simulink model "Experiment_cs"  (Simulink 8.8)
settings: Solver=ode5  StartTime=0.0  StopTime=inf  FixedStep=0.0005  RelTol=1e-3
PreLoadFcn:
  | check_NUTS_defined;
  | 
  | assignin('base',['model_closed_' bdroot],false);
InitFcn:
  | PreScanExperimentInitFcn(bdroot)
StopFcn:
  | PreScanExperimentStopFcn(bdroot)
undefined symbols (not defined in the file): DiscIntNeverNeededParam, FromPrescan, IdealSensors, psi, vd01, vd02, vd03, vd4, x, y
libraries: PreScanSimulinkLibrary x12, PreScanUsefulBlocks x8
(part 3 of 5)

== system Experiment_cs/Mazda_RX8_1/Dynamics_UserSpecified/SingleVehicle_01/VehicleDynamics ==
  VehicleStateLast : Inport
  accelCmd : Inport  Port=2
  brakeCmd : Inport  Port=3
  steerCmd : Inport  Port=4
  Bus Assignment : BusAssignment  AssignedSignals=x,y,psi
  Bus Selector : BusSelector  OutputSignals=x,y,z,u,v,w,theta,phi,psi
  F by m : Gain  Gain=1/veh_struct.mass*1000
  Integrator : Integrator  InitialCondition=veh_struct.init.u
  KinematicVehicleModel : MATLAB Function  TreatAsAtomicUnit=on
  MuxState : Subsystem  Tag=MuxState  mask(Empty Dynamics State Block){positioningmode=on, TimeStep=1/20}
      mask prompts: positioningmode "Positioning Mode"; TimeStep "Auto Assigned: Time Step [s]"
      mask help:
      | Build the state of an actor based on user input.
      | The user can either use positioning mode or dynamics mode.
      | - When using positioning mode the position and orientation of the actor are set directly based on the input. Expected input is relative to the initial position and orientation of the actor. It's also possible to specify the velocity of the actor, though this input isn't used, only passed on.
      | - When using dynamics mode the position input is ignored. Expected input is velocity and orientation. The velocity is relative the current orientation of the actor, while orientation is relative to its initial orientation. The position of the actor is calculated based on the velocity and orientation given.
      settings: DeleteFcn=PreScanBlockDeleteFcn;
  Scope : Scope
  Sum : Sum  Inputs=|++
  int_dX : Integrator  InitialCondition=veh_struct.init.X
  int_dY : Integrator  InitialCondition=veh_struct.init.Y
  int_dpsi : Integrator  InitialCondition=veh_struct.init.psi
  VehicleStateBus : Outport
  PrescanState : Outport  Port=2
  wires:
  int_dpsi/1 -> KinematicVehicleModel/3(psi), Bus Assignment/4
  int_dY/1 -> Bus Assignment/3
  int_dX/1 -> Bus Assignment/2
  KinematicVehicleModel/3(dpsi) -> int_dpsi/1
  KinematicVehicleModel/1(dX) -> int_dX/1
  KinematicVehicleModel/2(dY) -> int_dY/1
  Integrator/1 -> KinematicVehicleModel/1(u), Scope/1
  F by m/1 -> Integrator/1
  Sum/1 -> F by m/1
  brakeCmd/1 -> Sum/2
  accelCmd/1 -> Sum/1
  steerCmd/1 -> KinematicVehicleModel/2(delta)
  VehicleStateLast/1 -> Bus Assignment/1
  Bus Selector/8 -> MuxState/8(P [rad])  "<phi>"
  Bus Selector/9 -> MuxState/9(Y [rad])  "<psi>"
  Bus Selector/7 -> MuxState/7(R [rad])  "<theta>"
  Bus Selector/2 -> MuxState/2(y [m])  "<y>"
  Bus Selector/1 -> MuxState/1(x [m])  "<x>"
  Bus Selector/6 -> MuxState/6(dz [m/s])  "<w>"
  Bus Selector/5 -> MuxState/5(dy [m/s])  "<v>"
  Bus Selector/4 -> MuxState/4(dx [m/s])  "<u>"
  Bus Selector/3 -> MuxState/3(z [m])  "<z>"
  Bus Assignment/1 -> VehicleStateBus/1, Bus Selector/1
  MuxState/1(state) -> PrescanState/1

== system Experiment_cs/Mazda_RX8_1/SELF_Demux/compas converter/cart2compas ==
  Angle [deg] : Inport
  Constant : Constant  Value=90
  Constant1 : Constant  Value=360
  Gain : Gain  Gain=1/360
  Gain1 : Gain  Gain=360
  Gain2 : Gain  Gain=-1
  Rounding Function : Rounding
  Sum : Sum  Inputs=|-+
  Sum1 : Sum  Inputs=-+|
  Sum2 : Sum  Inputs=++|
  heading [deg] : Outport
  wires:
  Sum2/1 -> heading [deg]/1
  Constant1/1 -> Sum2/1
  Gain2/1 -> Sum2/2
  Constant/1 -> Sum1/1
  Sum1/1 -> Sum/2, Gain/1
  Sum/1 -> Gain2/1
  Angle [deg]/1 -> Sum1/2
  Gain1/1 -> Sum/1
  Rounding Function/1 -> Gain1/1
  Gain/1 -> Rounding Function/1

== system Experiment_cs/Toyota_Yaris_1/Dynamics_UserSpecified/SingleVehicle_01/Controller ==
  VehcileStateLast : Inport
  PrescanSimData : Inport  Port=2
  Trigger : TriggerPort  VariantControl=Variant  PortDimensions=1
  Actuation : Subsystem
  CollectSensorData : Subsystem
  CtlMainBusUnitDelayAndInit : Subsystem
  FeaturedFunctions : Subsystem
  SituationalAwareness : Subsystem
  StrategicArbitration : Subsystem
  accelCmd : Outport
  brakeCmd : Outport  Port=2
  steerCmd : Outport  Port=3
  ControllerMainBus : Outport  Port=4
  wires:
  CollectSensorData/2(IdealSensorBus) -> SituationalAwareness/2(IdealSensorBus)
  CollectSensorData/1(PrescanSimDataBus) -> SituationalAwareness/1(PrescanSimDataBus)
  CtlMainBusUnitDelayAndInit/1(CtlBusDelayed) -> CollectSensorData/3(ControllerMainBusIn)
  Actuation/4(ControllerMainBusOut) -> ControllerMainBus/1, CtlMainBusUnitDelayAndInit/1(CtlBus)
  VehcileStateLast/1 -> CollectSensorData/2(VehicleStateLast)
  CollectSensorData/3(ControllerMainBusOut) -> SituationalAwareness/3(ControllerMainBusIn)
  SituationalAwareness/2(ControllerMainBusOut) -> FeaturedFunctions/2(ControllerMainBusIn)
  SituationalAwareness/1(SituationBus) -> FeaturedFunctions/1(SituationBus)
  FeaturedFunctions/1(FeatureReqBus) -> StrategicArbitration/1(FeatureReqBus)
  FeaturedFunctions/2(ControllerMainBusOut) -> StrategicArbitration/2(ControllerMainBusIn)
  StrategicArbitration/2(ControllerMainBusOut) -> Actuation/2(ControllerMainBusIn)
  StrategicArbitration/1(ArbitratedActuationReq) -> Actuation/1(ArbitratedActuationReq)
  Actuation/3(steerCmd) -> steerCmd/1
  Actuation/2(brakeCmd) -> brakeCmd/1
  Actuation/1(accelCmd) -> accelCmd/1
  PrescanSimData/1 -> CollectSensorData/1(PreScanSimData)

== system Experiment_cs/Toyota_Yaris_1/Dynamics_UserSpecified/SingleVehicle_01/Monitor ==
  VehicleStateBus : Inport
  ControllerMainBus : Inport  Port=2
  ControllerMainBusStorage : Subsystem
  VehicleStateBusStorage : ToWorkspace  VariableName=vd02_DataVehicleBus  SaveFormat=Timeseries  SampleTime=-1
  wires:
  ControllerMainBus/1 -> ControllerMainBusStorage/1(ControllerMainBus)
  VehicleStateBus/1 -> VehicleStateBusStorage/1

== system Experiment_cs/Toyota_Yaris_1/Dynamics_UserSpecified/SingleVehicle_01/VehStateBusUnitDelayAndInit ==
  VehStateBus : Inport
  MATLAB Function : MATLAB Function  TreatAsAtomicUnit=on
  Memory : Memory  InheritSampleTime=on
  VehStateBusDelayed : Outport
  wires:
  MATLAB Function/1(y) -> VehStateBusDelayed/1
  VehStateBus/1 -> Memory/1
  Memory/1 -> MATLAB Function/1(u)

== system Experiment_cs/Toyota_Yaris_1/Dynamics_UserSpecified/SingleVehicle_01/VehicleDynamics ==
  VehicleStateLast : Inport
  accelCmd : Inport  Port=2
  brakeCmd : Inport  Port=3
  steerCmd : Inport  Port=4
  Bus Assignment : BusAssignment  AssignedSignals=x,y,psi
  Bus Selector : BusSelector  OutputSignals=x,y,z,u,v,w,theta,phi,psi
  F by m : Gain  Gain=1/veh_struct.mass*1000
  Integrator : Integrator  InitialCondition=veh_struct.init.u
  KinematicVehicleModel : MATLAB Function  TreatAsAtomicUnit=on
  MuxState : Subsystem  Tag=MuxState  mask(Empty Dynamics State Block){positioningmode=on, TimeStep=1/20}
      mask prompts: positioningmode "Positioning Mode"; TimeStep "Auto Assigned: Time Step [s]"
      mask help:
      | Build the state of an actor based on user input.
      | The user can either use positioning mode or dynamics mode.
      | - When using positioning mode the position and orientation of the actor are set directly based on the input. Expected input is relative to the initial position and orientation of the actor. It's also possible to specify the velocity of the actor, though this input isn't used, only passed on.
      | - When using dynamics mode the position input is ignored. Expected input is velocity and orientation. The velocity is relative the current orientation of the actor, while orientation is relative to its initial orientation. The position of the actor is calculated based on the velocity and orientation given.
      settings: DeleteFcn=PreScanBlockDeleteFcn;
  Scope : Scope
  Sum : Sum  Inputs=|++
  int_dX : Integrator  InitialCondition=veh_struct.init.X
  int_dY : Integrator  InitialCondition=veh_struct.init.Y
  int_dpsi : Integrator  InitialCondition=veh_struct.init.psi
  VehicleStateBus : Outport
  PrescanState : Outport  Port=2
  wires:
  int_dpsi/1 -> KinematicVehicleModel/3(psi), Bus Assignment/4
  int_dY/1 -> Bus Assignment/3
  int_dX/1 -> Bus Assignment/2
  KinematicVehicleModel/3(dpsi) -> int_dpsi/1
  KinematicVehicleModel/1(dX) -> int_dX/1
  KinematicVehicleModel/2(dY) -> int_dY/1
  Integrator/1 -> KinematicVehicleModel/1(u), Scope/1
  F by m/1 -> Integrator/1
  Sum/1 -> F by m/1
  brakeCmd/1 -> Sum/2
  accelCmd/1 -> Sum/1
  steerCmd/1 -> KinematicVehicleModel/2(delta)
  VehicleStateLast/1 -> Bus Assignment/1
  Bus Selector/8 -> MuxState/8(P [rad])  "<phi>"
  Bus Selector/9 -> MuxState/9(Y [rad])  "<psi>"
  Bus Selector/7 -> MuxState/7(R [rad])  "<theta>"
  Bus Selector/2 -> MuxState/2(y [m])  "<y>"
  Bus Selector/1 -> MuxState/1(x [m])  "<x>"
  Bus Selector/6 -> MuxState/6(dz [m/s])  "<w>"
  Bus Selector/5 -> MuxState/5(dy [m/s])  "<v>"
  Bus Selector/4 -> MuxState/4(dx [m/s])  "<u>"
  Bus Selector/3 -> MuxState/3(z [m])  "<z>"
  Bus Assignment/1 -> VehicleStateBus/1, Bus Selector/1
  MuxState/1(state) -> PrescanState/1

== system Experiment_cs/Toyota_Yaris_1/SELF_Demux/compas converter/cart2compas ==
  Angle [deg] : Inport
  Constant : Constant  Value=90
  Constant1 : Constant  Value=360
  Gain : Gain  Gain=1/360
  Gain1 : Gain  Gain=360
  Gain2 : Gain  Gain=-1
  Rounding Function : Rounding
  Sum : Sum  Inputs=|-+
  Sum1 : Sum  Inputs=-+|
  Sum2 : Sum  Inputs=++|
  heading [deg] : Outport
  wires:
  Sum2/1 -> heading [deg]/1
  Constant1/1 -> Sum2/1
  Gain2/1 -> Sum2/2
  Constant/1 -> Sum1/1
  Sum1/1 -> Sum/2, Gain/1
  Sum/1 -> Gain2/1
  Angle [deg]/1 -> Sum1/2
  Gain1/1 -> Sum/1
  Rounding Function/1 -> Gain1/1
  Gain/1 -> Rounding Function/1

== system Experiment_cs/Actros_2541_1/Dynamics_UserSpecified/SingleVehicle_01/Controller/Actuation ==
  ArbitratedActuationReq : Inport
  ControllerMainBusIn : Inport  Port=2
  ActuatorDrivers : MATLAB Function  TreatAsAtomicUnit=on
  Bus Assignment : BusAssignment  AssignedSignals=ActuationCmdBus
  Bus Selector : BusSelector  OutputSignals=ActuationCmdBus
  DynamicControls : MATLAB Function  TreatAsAtomicUnit=on
  accelCmd : Outport
  brakeCmd : Outport  Port=2
  steerCmd : Outport  Port=3
  ControllerMainBusOut : Outport  Port=4
  wires:
  ActuatorDrivers/3(steering_cmd) -> steerCmd/1
  ActuatorDrivers/1(accel_cmd) -> accelCmd/1
  ActuatorDrivers/2(decel_cmd) -> brakeCmd/1
  Bus Assignment/1 -> ControllerMainBusOut/1
  DynamicControls/1(ActCmds) -> Bus Assignment/2, ActuatorDrivers/1(ActCmds)
  Bus Selector/1 -> DynamicControls/3(ActCmdsPrev)  "<ActuationCmdBus>"
  ArbitratedActuationReq/1 -> DynamicControls/1(ActReq)
  ControllerMainBusIn/1 -> Bus Selector/1, Bus Assignment/1, DynamicControls/2(Ctl)

== system Experiment_cs/Actros_2541_1/Dynamics_UserSpecified/SingleVehicle_01/Controller/CollectSensorData ==
  PreScanSimData : Inport
  VehicleStateLast : Inport  Port=2
  ControllerMainBusIn : Inport  Port=3
  Bus Assignment : BusAssignment  AssignedSignals=FromPrescan,IdealSensors
  IdealSensorsProcess : Subsystem
  PrescanProcess : Subsystem
  PrescanSimDataBus : Outport
  IdealSensorBus : Outport  Port=2
  ControllerMainBusOut : Outport  Port=3
  wires:
  ControllerMainBusIn/1 -> Bus Assignment/1
  Bus Assignment/1 -> ControllerMainBusOut/1
  IdealSensorsProcess/1(IdealSensorsBus) -> Bus Assignment/3, IdealSensorBus/1
  VehicleStateLast/1 -> IdealSensorsProcess/1(VehicleState)
  PrescanProcess/1(PrescanSimDataBus) -> PrescanSimDataBus/1, Bus Assignment/2
  PreScanSimData/1 -> PrescanProcess/1(PrescanSimData)

== system Experiment_cs/Actros_2541_1/Dynamics_UserSpecified/SingleVehicle_01/Controller/CtlMainBusUnitDelayAndInit ==
  CtlBus : Inport
  MATLAB Function : MATLAB Function  TreatAsAtomicUnit=on
  Memory : Memory  InheritSampleTime=on
  CtlBusDelayed : Outport
  wires:
  MATLAB Function/1(y) -> CtlBusDelayed/1
  CtlBus/1 -> Memory/1
  Memory/1 -> MATLAB Function/1(u)

== system Experiment_cs/Actros_2541_1/Dynamics_UserSpecified/SingleVehicle_01/Controller/FeaturedFunctions ==
  SituationBus : Inport
  ControllerMainBusIn : Inport  Port=2
  Bus Assignment : BusAssignment  AssignedSignals=wpFollower
  Bus Assignment1 : BusAssignment  AssignedSignals=FunctionFeatures
  Bus Assignment2 : BusAssignment  AssignedSignals=situationBus
  Bus Selector : BusSelector  OutputSignals=FunctionFeatures
  Bus Selector2 : BusSelector  OutputSignals=FunctionFeatures.wpFollower
  wpFollower : MATLAB Function  TreatAsAtomicUnit=on
  FeatureReqBus : Outport
  ControllerMainBusOut : Outport  Port=2
  wires:
  Bus Selector2/1 -> wpFollower/1(prevWpAction)  "<wpFollower>"
  Bus Assignment2/1 -> ControllerMainBusOut/1
  wpFollower/2(newSituation) -> Bus Assignment2/2
  Bus Assignment1/1 -> Bus Assignment2/1
  Bus Assignment/1 -> FeatureReqBus/1, Bus Assignment1/2
  wpFollower/1(wpAction) -> Bus Assignment/2
  Bus Selector/1 -> Bus Assignment/1  "<FunctionFeatures>"
  SituationBus/1 -> wpFollower/2(prevSituation)
  ControllerMainBusIn/1 -> Bus Assignment1/1, Bus Selector2/1, Bus Selector/1

== system Experiment_cs/Actros_2541_1/Dynamics_UserSpecified/SingleVehicle_01/Controller/SituationalAwareness ==
  PrescanSimDataBus : Inport
  IdealSensorBus : Inport  Port=2
  ControllerMainBusIn : Inport  Port=3
  Bus Assignment : BusAssignment  AssignedSignals=situationBus
  Bus Selector : BusSelector  OutputSignals=situationBus
  situationAwareness : MATLAB Function  TreatAsAtomicUnit=on
  SituationBus : Outport
  ControllerMainBusOut : Outport  Port=2
  wires:
  Bus Assignment/1 -> ControllerMainBusOut/1
  situationAwareness/1(newSituation) -> SituationBus/1, Bus Assignment/2
  IdealSensorBus/1 -> situationAwareness/3(idealSensors)
  PrescanSimDataBus/1 -> situationAwareness/2(prescanSimData)
  Bus Selector/1 -> situationAwareness/1(prevSituation)  "<situationBus>"
  ControllerMainBusIn/1 -> Bus Selector/1, Bus Assignment/1

== system Experiment_cs/Actros_2541_1/Dynamics_UserSpecified/SingleVehicle_01/Controller/StrategicArbitration ==
  FeatureReqBus : Inport
  ControllerMainBusIn : Inport  Port=2
  Arbitration : MATLAB Function  TreatAsAtomicUnit=on
  Bus Assignment : BusAssignment  AssignedSignals=ArbitratedActuationReq
  ArbitratedActuationReq : Outport
  ControllerMainBusOut : Outport  Port=2
  wires:
  Bus Assignment/1 -> ControllerMainBusOut/1
  Arbitration/1(ArbitratedReq) -> ArbitratedActuationReq/1, Bus Assignment/2
  FeatureReqBus/1 -> Arbitration/1(FunctionFeatures)
  ControllerMainBusIn/1 -> Bus Assignment/1

== system Experiment_cs/Actros_2541_1/Dynamics_UserSpecified/SingleVehicle_01/Monitor/ControllerMainBusStorage ==
  ControllerMainBus : Inport
  ArbitratedActuationReqStorage : ToWorkspace  VariableName=vd4_DataControllerMain_ArbitrationActuationReq  SaveFormat=Timeseries  SampleTime=-1
  Bus Selector : BusSelector  OutputSignals=ArbitratedActuationReq,FunctionFeatures.wpFollower,situationBus.wP.finalWayPoint,situationBus.wP.currentWayPoint,situationBus.wP.wayPointArray,situationBus.selfAwarenessBus,IdealSensors,FromPrescan
  FromPrescanStorage : ToWorkspace  VariableName=vd4_DataControllerMain_FromPrescan  SaveFormat=Timeseries  SampleTime=-1
  Ground_1 : Ground
  IdealSensorsStorage : ToWorkspace  VariableName=vd4_DataControllerMain_IdealSensors  SaveFormat=Timeseries  SampleTime=-1
  Terminator_1 : Terminator
  currentWayPointStorage : ToWorkspace  VariableName=vd4_DataControllerMain_currentWayPoint  SaveFormat=Timeseries  SampleTime=-1
  finalWayPointStorarge : ToWorkspace  VariableName=vd4_DataControllerMain_finalWayPoint  SaveFormat=Timeseries  SampleTime=-1
  selfAwareessBusStorage : ToWorkspace  VariableName=vd4_DataControllerMain_selfAwareessBus  SaveFormat=Timeseries  SampleTime=-1
  wayPointArrayStorage : ToWorkspace  VariableName=vd4_DataControllerMain_wayPointArray  SampleTime=-1
  wpFollowerStorage : ToWorkspace  VariableName=vd4_DataControllerMain_wpFollower  SaveFormat=Timeseries  SampleTime=-1
  wires:
  Bus Selector/7 -> IdealSensorsStorage/1  "<IdealSensors>"
  Bus Selector/4 -> currentWayPointStorage/1  "<currentWayPoint>"
  Bus Selector/6 -> selfAwareessBusStorage/1  "<selfAwarenessBus>"
  Bus Selector/8 -> FromPrescanStorage/1  "<FromPrescan>"
  Bus Selector/3 -> finalWayPointStorarge/1  "<finalWayPoint>"
  Bus Selector/2 -> wpFollowerStorage/1  "<wpFollower>"
  Bus Selector/1 -> ArbitratedActuationReqStorage/1  "<ArbitratedActuationReq>"
  ControllerMainBus/1 -> Bus Selector/1
  Bus Selector/5 -> Terminator_1/1  "<wayPointArray>"
  Ground_1/1 -> wayPointArrayStorage/1

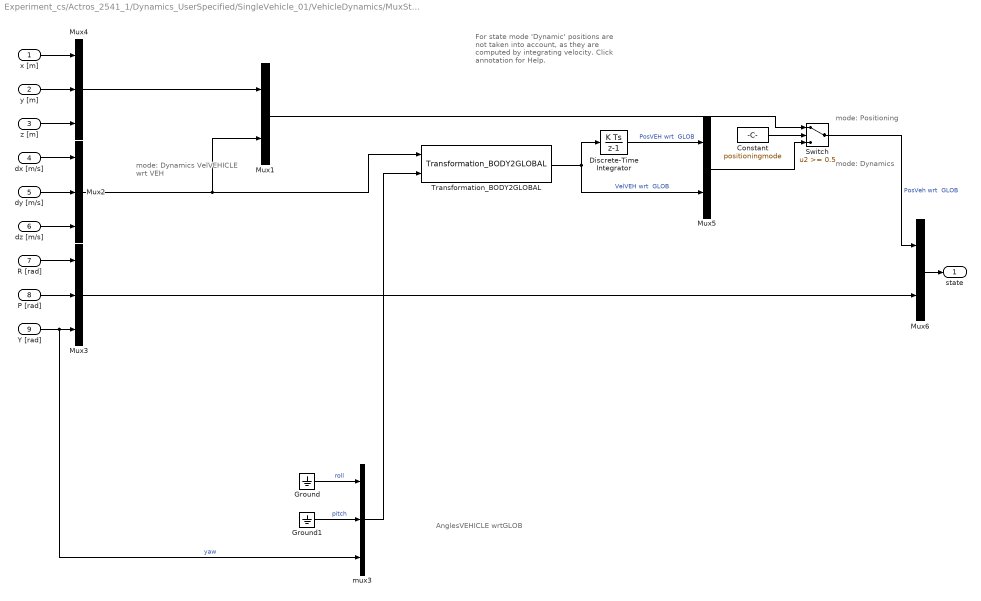
== system Experiment_cs/Actros_2541_1/Dynamics_UserSpecified/SingleVehicle_01/VehicleDynamics/MuxState ==
  note: For state mode 'Dynamic' positions
      | are not taken into account, as they
      | are computed by integrating velocity.
      | Click annotation for Help.
  note: AnglesVEHICLE
      | wrtGLOB
  note: mode: Dynamics
      | VelVEHICLE
      | wrt VEH
  note: mode: Positioning
  note: mode: Dynamics
  x [m] : Inport  SampleTime=TimeStep
  y [m] : Inport  Port=2  SampleTime=TimeStep
  z [m] : Inport  Port=3  SampleTime=TimeStep
  dx [m/s] : Inport  Port=4  SampleTime=TimeStep
  dy [m/s] : Inport  Port=5  SampleTime=TimeStep
  dz [m/s] : Inport  Port=6  SampleTime=TimeStep
  R [rad] : Inport  Port=7  SampleTime=TimeStep
  P [rad] : Inport  Port=8  SampleTime=TimeStep
  Y [rad] : Inport  Port=9  SampleTime=TimeStep
  Constant : Constant  DisableCoverage=on  Value=positioningmode
  Discrete-Time Integrator : DiscreteIntegrator  SampleTime=TimeStep  ICPrevOutput=DiscIntNeverNeededParam  ICPrevScaledInput=DiscIntNeverNeededParam
  Ground : Ground
  Ground1 : Ground
  Mux1 : Mux  Inputs=[3 3]
  Mux2 : Mux  Inputs=3
  Mux3 : Mux  Inputs=3
  Mux4 : Mux  Inputs=3
  Mux5 : Mux  Inputs=[3 3]
  Mux6 : Mux  Inputs=[6 3]
  Switch : Switch  Threshold=0.5
  Transformation_BODY2GLOBAL : PreScanSimulinkLibrary/Simple_Vehicle_Dynamics/Chassis/MuxDynState/Transformation_BODY2GLOBAL
  mux3 : Mux  Inputs=3
  state : Outport
  wires:
  Discrete-Time Integrator/1 -> Mux5/1  "PosVEH wrt  GLOB"
  Mux2/1 -> Transformation_BODY2GLOBAL/1, Mux1/2
  Ground/1 -> mux3/1  "roll"
  mux3/1 -> Transformation_BODY2GLOBAL/2
  Transformation_BODY2GLOBAL/1 -> Mux5/2, Discrete-Time Integrator/1  "VelVEH wrt  GLOB"
  Mux3/1 -> Mux6/2
  Y [rad]/1 -> Mux3/3, mux3/3  "yaw"
  Ground1/1 -> mux3/2  "pitch"
  x [m]/1 -> Mux4/1
  y [m]/1 -> Mux4/2
  z [m]/1 -> Mux4/3
  dx [m/s]/1 -> Mux2/1
  dy [m/s]/1 -> Mux2/2
  dz [m/s]/1 -> Mux2/3
  R [rad]/1 -> Mux3/1
  P [rad]/1 -> Mux3/2
  Switch/1 -> Mux6/1  "PosVeh wrt  GLOB"
  Mux1/1 -> Switch/1
  Mux5/1 -> Switch/3
  Mux4/1 -> Mux1/1
  Mux6/1 -> state/1
  Constant/1 -> Switch/2

== system Experiment_cs/Audi_A8_1/Dynamics_UserSpecified/SingleVehicle_01/Controller/Actuation ==
  ArbitratedActuationReq : Inport
  ControllerMainBusIn : Inport  Port=2
  ActuatorDrivers : MATLAB Function  TreatAsAtomicUnit=on
  Bus Assignment : BusAssignment  AssignedSignals=ActuationCmdBus
  Bus Selector : BusSelector  OutputSignals=ActuationCmdBus
  DynamicControls : MATLAB Function  TreatAsAtomicUnit=on
  accelCmd : Outport
  brakeCmd : Outport  Port=2
  steerCmd : Outport  Port=3
  ControllerMainBusOut : Outport  Port=4
  wires:
  ActuatorDrivers/3(steering_cmd) -> steerCmd/1
  ActuatorDrivers/1(accel_cmd) -> accelCmd/1
  ActuatorDrivers/2(decel_cmd) -> brakeCmd/1
  Bus Assignment/1 -> ControllerMainBusOut/1
  DynamicControls/1(ActCmds) -> Bus Assignment/2, ActuatorDrivers/1(ActCmds)
  Bus Selector/1 -> DynamicControls/3(ActCmdsPrev)  "<ActuationCmdBus>"
  ArbitratedActuationReq/1 -> DynamicControls/1(ActReq)
  ControllerMainBusIn/1 -> Bus Selector/1, Bus Assignment/1, DynamicControls/2(Ctl)

== system Experiment_cs/Audi_A8_1/Dynamics_UserSpecified/SingleVehicle_01/Controller/CollectSensorData ==
  PreScanSimData : Inport
  VehicleStateLast : Inport  Port=2
  ControllerMainBusIn : Inport  Port=3
  Bus Assignment : BusAssignment  AssignedSignals=FromPrescan,IdealSensors
  IdealSensorsProcess : Subsystem
  PrescanProcess : Subsystem
  PrescanSimDataBus : Outport
  IdealSensorBus : Outport  Port=2
  ControllerMainBusOut : Outport  Port=3
  wires:
  ControllerMainBusIn/1 -> Bus Assignment/1
  Bus Assignment/1 -> ControllerMainBusOut/1
  IdealSensorsProcess/1(IdealSensorsBus) -> Bus Assignment/3, IdealSensorBus/1
  VehicleStateLast/1 -> IdealSensorsProcess/1(VehicleState)
  PrescanProcess/1(PrescanSimDataBus) -> PrescanSimDataBus/1, Bus Assignment/2
  PreScanSimData/1 -> PrescanProcess/1(PrescanSimData)

== system Experiment_cs/Audi_A8_1/Dynamics_UserSpecified/SingleVehicle_01/Controller/CtlMainBusUnitDelayAndInit ==
  CtlBus : Inport
  MATLAB Function : MATLAB Function  TreatAsAtomicUnit=on
  Memory : Memory  InheritSampleTime=on
  CtlBusDelayed : Outport
  wires:
  MATLAB Function/1(y) -> CtlBusDelayed/1
  CtlBus/1 -> Memory/1
  Memory/1 -> MATLAB Function/1(u)

== system Experiment_cs/Audi_A8_1/Dynamics_UserSpecified/SingleVehicle_01/Controller/FeaturedFunctions ==
  SituationBus : Inport
  ControllerMainBusIn : Inport  Port=2
  Bus Assignment : BusAssignment  AssignedSignals=wpFollower
  Bus Assignment1 : BusAssignment  AssignedSignals=FunctionFeatures
  Bus Assignment2 : BusAssignment  AssignedSignals=situationBus
  Bus Selector : BusSelector  OutputSignals=FunctionFeatures
  Bus Selector2 : BusSelector  OutputSignals=FunctionFeatures.wpFollower
  wpFollower : MATLAB Function  TreatAsAtomicUnit=on
  FeatureReqBus : Outport
  ControllerMainBusOut : Outport  Port=2
  wires:
  Bus Selector2/1 -> wpFollower/1(prevWpAction)  "<wpFollower>"
  Bus Assignment2/1 -> ControllerMainBusOut/1
  wpFollower/2(newSituation) -> Bus Assignment2/2
  Bus Assignment1/1 -> Bus Assignment2/1
  Bus Assignment/1 -> FeatureReqBus/1, Bus Assignment1/2
  wpFollower/1(wpAction) -> Bus Assignment/2
  Bus Selector/1 -> Bus Assignment/1  "<FunctionFeatures>"
  SituationBus/1 -> wpFollower/2(prevSituation)
  ControllerMainBusIn/1 -> Bus Assignment1/1, Bus Selector2/1, Bus Selector/1

== system Experiment_cs/Audi_A8_1/Dynamics_UserSpecified/SingleVehicle_01/Controller/SituationalAwareness ==
  PrescanSimDataBus : Inport
  IdealSensorBus : Inport  Port=2
  ControllerMainBusIn : Inport  Port=3
  Bus Assignment : BusAssignment  AssignedSignals=situationBus
  Bus Selector : BusSelector  OutputSignals=situationBus
  situationAwareness : MATLAB Function  TreatAsAtomicUnit=on
  SituationBus : Outport
  ControllerMainBusOut : Outport  Port=2
  wires:
  Bus Assignment/1 -> ControllerMainBusOut/1
  situationAwareness/1(newSituation) -> SituationBus/1, Bus Assignment/2
  IdealSensorBus/1 -> situationAwareness/3(idealSensors)
  PrescanSimDataBus/1 -> situationAwareness/2(prescanSimData)
  Bus Selector/1 -> situationAwareness/1(prevSituation)  "<situationBus>"
  ControllerMainBusIn/1 -> Bus Selector/1, Bus Assignment/1

== system Experiment_cs/Audi_A8_1/Dynamics_UserSpecified/SingleVehicle_01/Controller/StrategicArbitration ==
  FeatureReqBus : Inport
  ControllerMainBusIn : Inport  Port=2
  Arbitration : MATLAB Function  TreatAsAtomicUnit=on
  Bus Assignment : BusAssignment  AssignedSignals=ArbitratedActuationReq
  ArbitratedActuationReq : Outport
  ControllerMainBusOut : Outport  Port=2
  wires:
  Bus Assignment/1 -> ControllerMainBusOut/1
  Arbitration/1(ArbitratedReq) -> ArbitratedActuationReq/1, Bus Assignment/2
  FeatureReqBus/1 -> Arbitration/1(FunctionFeatures)
  ControllerMainBusIn/1 -> Bus Assignment/1

== system Experiment_cs/Audi_A8_1/Dynamics_UserSpecified/SingleVehicle_01/Monitor/ControllerMainBusStorage ==
  ControllerMainBus : Inport
  ArbitratedActuationReqStorage : ToWorkspace  VariableName=vd03_DataControllerMain_ArbitrationActuationReq  SaveFormat=Timeseries  SampleTime=-1
  Bus Selector : BusSelector  OutputSignals=ArbitratedActuationReq,FunctionFeatures.wpFollower,situationBus.wP.finalWayPoint,situationBus.wP.currentWayPoint,situationBus.wP.wayPointArray,situationBus.selfAwarenessBus,IdealSensors,FromPrescan
  FromPrescanStorage : ToWorkspace  VariableName=vd03_DataControllerMain_FromPrescan  SaveFormat=Timeseries  SampleTime=-1
  Ground_1 : Ground
  IdealSensorsStorage : ToWorkspace  VariableName=vd03_DataControllerMain_IdealSensors  SaveFormat=Timeseries  SampleTime=-1
  Terminator_1 : Terminator
  currentWayPointStorage : ToWorkspace  VariableName=vd03_DataControllerMain_currentWayPoint  SaveFormat=Timeseries  SampleTime=-1
  finalWayPointStorarge : ToWorkspace  VariableName=vd03_DataControllerMain_finalWayPoint  SaveFormat=Timeseries  SampleTime=-1
  selfAwareessBusStorage : ToWorkspace  VariableName=vd03_DataControllerMain_selfAwareessBus  SaveFormat=Timeseries  SampleTime=-1
  wayPointArrayStorage : ToWorkspace  VariableName=vd03_DataControllerMain_wayPointArray  SampleTime=-1
  wpFollowerStorage : ToWorkspace  VariableName=vd03_DataControllerMain_wpFollower  SaveFormat=Timeseries  SampleTime=-1
  wires:
  Bus Selector/7 -> IdealSensorsStorage/1  "<IdealSensors>"
  Bus Selector/4 -> currentWayPointStorage/1  "<currentWayPoint>"
  Bus Selector/6 -> selfAwareessBusStorage/1  "<selfAwarenessBus>"
  Bus Selector/8 -> FromPrescanStorage/1  "<FromPrescan>"
  Bus Selector/3 -> finalWayPointStorarge/1  "<finalWayPoint>"
  Bus Selector/2 -> wpFollowerStorage/1  "<wpFollower>"
  Bus Selector/1 -> ArbitratedActuationReqStorage/1  "<ArbitratedActuationReq>"
  ControllerMainBus/1 -> Bus Selector/1
  Bus Selector/5 -> Terminator_1/1  "<wayPointArray>"
  Ground_1/1 -> wayPointArrayStorage/1

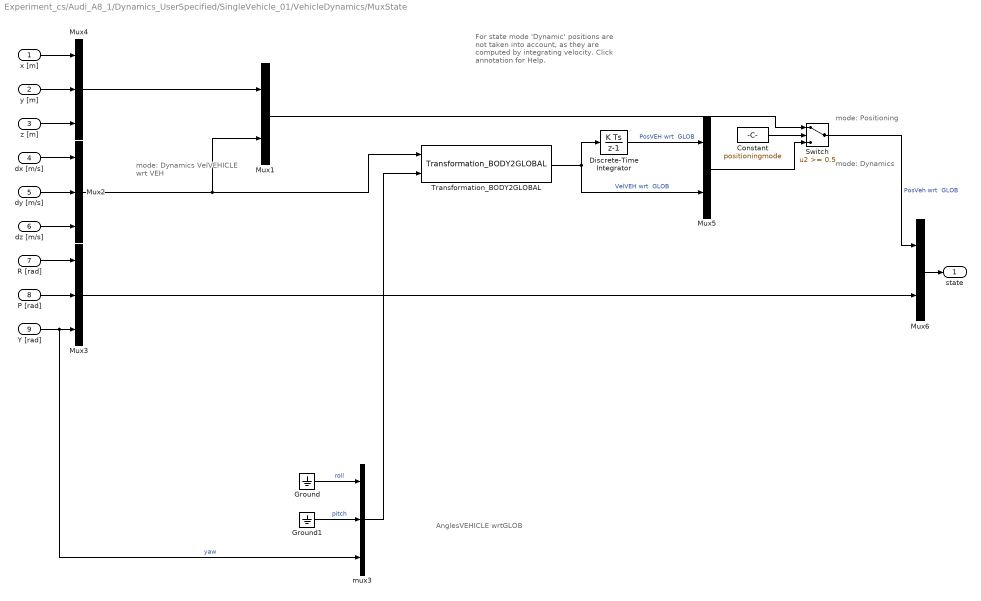
== system Experiment_cs/Audi_A8_1/Dynamics_UserSpecified/SingleVehicle_01/VehicleDynamics/MuxState ==
  note: For state mode 'Dynamic' positions
      | are not taken into account, as they
      | are computed by integrating velocity.
      | Click annotation for Help.
  note: AnglesVEHICLE
      | wrtGLOB
  note: mode: Dynamics
      | VelVEHICLE
      | wrt VEH
  note: mode: Positioning
  note: mode: Dynamics
  x [m] : Inport  SampleTime=TimeStep
  y [m] : Inport  Port=2  SampleTime=TimeStep
  z [m] : Inport  Port=3  SampleTime=TimeStep
  dx [m/s] : Inport  Port=4  SampleTime=TimeStep
  dy [m/s] : Inport  Port=5  SampleTime=TimeStep
  dz [m/s] : Inport  Port=6  SampleTime=TimeStep
  R [rad] : Inport  Port=7  SampleTime=TimeStep
  P [rad] : Inport  Port=8  SampleTime=TimeStep
  Y [rad] : Inport  Port=9  SampleTime=TimeStep
  Constant : Constant  DisableCoverage=on  Value=positioningmode
  Discrete-Time Integrator : DiscreteIntegrator  SampleTime=TimeStep  ICPrevOutput=DiscIntNeverNeededParam  ICPrevScaledInput=DiscIntNeverNeededParam
  Ground : Ground
  Ground1 : Ground
  Mux1 : Mux  Inputs=[3 3]
  Mux2 : Mux  Inputs=3
  Mux3 : Mux  Inputs=3
  Mux4 : Mux  Inputs=3
  Mux5 : Mux  Inputs=[3 3]
  Mux6 : Mux  Inputs=[6 3]
  Switch : Switch  Threshold=0.5
  Transformation_BODY2GLOBAL : PreScanSimulinkLibrary/Simple_Vehicle_Dynamics/Chassis/MuxDynState/Transformation_BODY2GLOBAL
  mux3 : Mux  Inputs=3
  state : Outport
  wires:
  Discrete-Time Integrator/1 -> Mux5/1  "PosVEH wrt  GLOB"
  Mux2/1 -> Transformation_BODY2GLOBAL/1, Mux1/2
  Ground/1 -> mux3/1  "roll"
  mux3/1 -> Transformation_BODY2GLOBAL/2
  Transformation_BODY2GLOBAL/1 -> Mux5/2, Discrete-Time Integrator/1  "VelVEH wrt  GLOB"
  Mux3/1 -> Mux6/2
  Y [rad]/1 -> Mux3/3, mux3/3  "yaw"
  Ground1/1 -> mux3/2  "pitch"
  x [m]/1 -> Mux4/1
  y [m]/1 -> Mux4/2
  z [m]/1 -> Mux4/3
  dx [m/s]/1 -> Mux2/1
  dy [m/s]/1 -> Mux2/2
  dz [m/s]/1 -> Mux2/3
  R [rad]/1 -> Mux3/1
  P [rad]/1 -> Mux3/2
  Switch/1 -> Mux6/1  "PosVeh wrt  GLOB"
  Mux1/1 -> Switch/1
  Mux5/1 -> Switch/3
  Mux4/1 -> Mux1/1
  Mux6/1 -> state/1
  Constant/1 -> Switch/2

== system Experiment_cs/Mazda_RX8_1/Dynamics_UserSpecified/SingleVehicle_01/Controller/Actuation ==
  ArbitratedActuationReq : Inport
  ControllerMainBusIn : Inport  Port=2
  ActuatorDrivers : MATLAB Function  TreatAsAtomicUnit=on
  Bus Assignment : BusAssignment  AssignedSignals=ActuationCmdBus
  Bus Selector : BusSelector  OutputSignals=ActuationCmdBus
  DynamicControls : MATLAB Function  TreatAsAtomicUnit=on
  accelCmd : Outport
  brakeCmd : Outport  Port=2
  steerCmd : Outport  Port=3
  ControllerMainBusOut : Outport  Port=4
  wires:
  ActuatorDrivers/3(steering_cmd) -> steerCmd/1
  ActuatorDrivers/1(accel_cmd) -> accelCmd/1
  ActuatorDrivers/2(decel_cmd) -> brakeCmd/1
  Bus Assignment/1 -> ControllerMainBusOut/1
  DynamicControls/1(ActCmds) -> Bus Assignment/2, ActuatorDrivers/1(ActCmds)
  Bus Selector/1 -> DynamicControls/3(ActCmdsPrev)  "<ActuationCmdBus>"
  ArbitratedActuationReq/1 -> DynamicControls/1(ActReq)
  ControllerMainBusIn/1 -> Bus Selector/1, Bus Assignment/1, DynamicControls/2(Ctl)

== system Experiment_cs/Mazda_RX8_1/Dynamics_UserSpecified/SingleVehicle_01/Controller/CollectSensorData ==
  PreScanSimData : Inport
  VehicleStateLast : Inport  Port=2
  ControllerMainBusIn : Inport  Port=3
  Bus Assignment : BusAssignment  AssignedSignals=FromPrescan,IdealSensors
  IdealSensorsProcess : Subsystem
  PrescanProcess : Subsystem
  PrescanSimDataBus : Outport
  IdealSensorBus : Outport  Port=2
  ControllerMainBusOut : Outport  Port=3
  wires:
  ControllerMainBusIn/1 -> Bus Assignment/1
  Bus Assignment/1 -> ControllerMainBusOut/1
  IdealSensorsProcess/1(IdealSensorsBus) -> Bus Assignment/3, IdealSensorBus/1
  VehicleStateLast/1 -> IdealSensorsProcess/1(VehicleState)
  PrescanProcess/1(PrescanSimDataBus) -> PrescanSimDataBus/1, Bus Assignment/2
  PreScanSimData/1 -> PrescanProcess/1(PrescanSimData)

== system Experiment_cs/Mazda_RX8_1/Dynamics_UserSpecified/SingleVehicle_01/Controller/CtlMainBusUnitDelayAndInit ==
  CtlBus : Inport
  MATLAB Function : MATLAB Function  TreatAsAtomicUnit=on
  Memory : Memory  InheritSampleTime=on
  CtlBusDelayed : Outport
  wires:
  MATLAB Function/1(y) -> CtlBusDelayed/1
  CtlBus/1 -> Memory/1
  Memory/1 -> MATLAB Function/1(u)

== system Experiment_cs/Mazda_RX8_1/Dynamics_UserSpecified/SingleVehicle_01/Controller/FeaturedFunctions ==
  SituationBus : Inport
  ControllerMainBusIn : Inport  Port=2
  Bus Assignment : BusAssignment  AssignedSignals=wpFollower
  Bus Assignment1 : BusAssignment  AssignedSignals=FunctionFeatures
  Bus Assignment2 : BusAssignment  AssignedSignals=situationBus
  Bus Selector : BusSelector  OutputSignals=FunctionFeatures
  Bus Selector2 : BusSelector  OutputSignals=FunctionFeatures.wpFollower
  wpFollower : MATLAB Function  TreatAsAtomicUnit=on
  FeatureReqBus : Outport
  ControllerMainBusOut : Outport  Port=2
  wires:
  Bus Selector2/1 -> wpFollower/1(prevWpAction)  "<wpFollower>"
  Bus Assignment2/1 -> ControllerMainBusOut/1
  wpFollower/2(newSituation) -> Bus Assignment2/2
  Bus Assignment1/1 -> Bus Assignment2/1
  Bus Assignment/1 -> FeatureReqBus/1, Bus Assignment1/2
  wpFollower/1(wpAction) -> Bus Assignment/2
  Bus Selector/1 -> Bus Assignment/1  "<FunctionFeatures>"
  SituationBus/1 -> wpFollower/2(prevSituation)
  ControllerMainBusIn/1 -> Bus Assignment1/1, Bus Selector2/1, Bus Selector/1

== system Experiment_cs/Mazda_RX8_1/Dynamics_UserSpecified/SingleVehicle_01/Controller/SituationalAwareness ==
  PrescanSimDataBus : Inport
  IdealSensorBus : Inport  Port=2
  ControllerMainBusIn : Inport  Port=3
  Bus Assignment : BusAssignment  AssignedSignals=situationBus
  Bus Selector : BusSelector  OutputSignals=situationBus
  situationAwareness : MATLAB Function  TreatAsAtomicUnit=on
  SituationBus : Outport
  ControllerMainBusOut : Outport  Port=2
  wires:
  Bus Assignment/1 -> ControllerMainBusOut/1
  situationAwareness/1(newSituation) -> SituationBus/1, Bus Assignment/2
  IdealSensorBus/1 -> situationAwareness/3(idealSensors)
  PrescanSimDataBus/1 -> situationAwareness/2(prescanSimData)
  Bus Selector/1 -> situationAwareness/1(prevSituation)  "<situationBus>"
  ControllerMainBusIn/1 -> Bus Selector/1, Bus Assignment/1

== system Experiment_cs/Mazda_RX8_1/Dynamics_UserSpecified/SingleVehicle_01/Controller/StrategicArbitration ==
  FeatureReqBus : Inport
  ControllerMainBusIn : Inport  Port=2
  Arbitration : MATLAB Function  TreatAsAtomicUnit=on
  Bus Assignment : BusAssignment  AssignedSignals=ArbitratedActuationReq
  ArbitratedActuationReq : Outport
  ControllerMainBusOut : Outport  Port=2
  wires:
  Bus Assignment/1 -> ControllerMainBusOut/1
  Arbitration/1(ArbitratedReq) -> ArbitratedActuationReq/1, Bus Assignment/2
  FeatureReqBus/1 -> Arbitration/1(FunctionFeatures)
  ControllerMainBusIn/1 -> Bus Assignment/1

== system Experiment_cs/Mazda_RX8_1/Dynamics_UserSpecified/SingleVehicle_01/Monitor/ControllerMainBusStorage ==
  ControllerMainBus : Inport
  ArbitratedActuationReqStorage : ToWorkspace  VariableName=vd01_DataControllerMain_ArbitrationActuationReq  SaveFormat=Timeseries  SampleTime=-1
  Bus Selector : BusSelector  OutputSignals=ArbitratedActuationReq,FunctionFeatures.wpFollower,situationBus.wP.finalWayPoint,situationBus.wP.currentWayPoint,situationBus.wP.wayPointArray,situationBus.selfAwarenessBus,IdealSensors,FromPrescan
  FromPrescanStorage : ToWorkspace  VariableName=vd01_DataControllerMain_FromPrescan  SaveFormat=Timeseries  SampleTime=-1
  Ground_1 : Ground
  IdealSensorsStorage : ToWorkspace  VariableName=vd01_DataControllerMain_IdealSensors  SaveFormat=Timeseries  SampleTime=-1
  Terminator_1 : Terminator
  currentWayPointStorage : ToWorkspace  VariableName=vd01_DataControllerMain_currentWayPoint  SaveFormat=Timeseries  SampleTime=-1
  finalWayPointStorarge : ToWorkspace  VariableName=vd01_DataControllerMain_finalWayPoint  SaveFormat=Timeseries  SampleTime=-1
  selfAwareessBusStorage : ToWorkspace  VariableName=vd01_DataControllerMain_selfAwareessBus  SaveFormat=Timeseries  SampleTime=-1
  wayPointArrayStorage : ToWorkspace  VariableName=vd01_DataControllerMain_wayPointArray  SampleTime=-1
  wpFollowerStorage : ToWorkspace  VariableName=vd01_DataControllerMain_wpFollower  SaveFormat=Timeseries  SampleTime=-1
  wires:
  Bus Selector/7 -> IdealSensorsStorage/1  "<IdealSensors>"
  Bus Selector/4 -> currentWayPointStorage/1  "<currentWayPoint>"
  Bus Selector/6 -> selfAwareessBusStorage/1  "<selfAwarenessBus>"
  Bus Selector/8 -> FromPrescanStorage/1  "<FromPrescan>"
  Bus Selector/3 -> finalWayPointStorarge/1  "<finalWayPoint>"
  Bus Selector/2 -> wpFollowerStorage/1  "<wpFollower>"
  Bus Selector/1 -> ArbitratedActuationReqStorage/1  "<ArbitratedActuationReq>"
  ControllerMainBus/1 -> Bus Selector/1
  Bus Selector/5 -> Terminator_1/1  "<wayPointArray>"
  Ground_1/1 -> wayPointArrayStorage/1

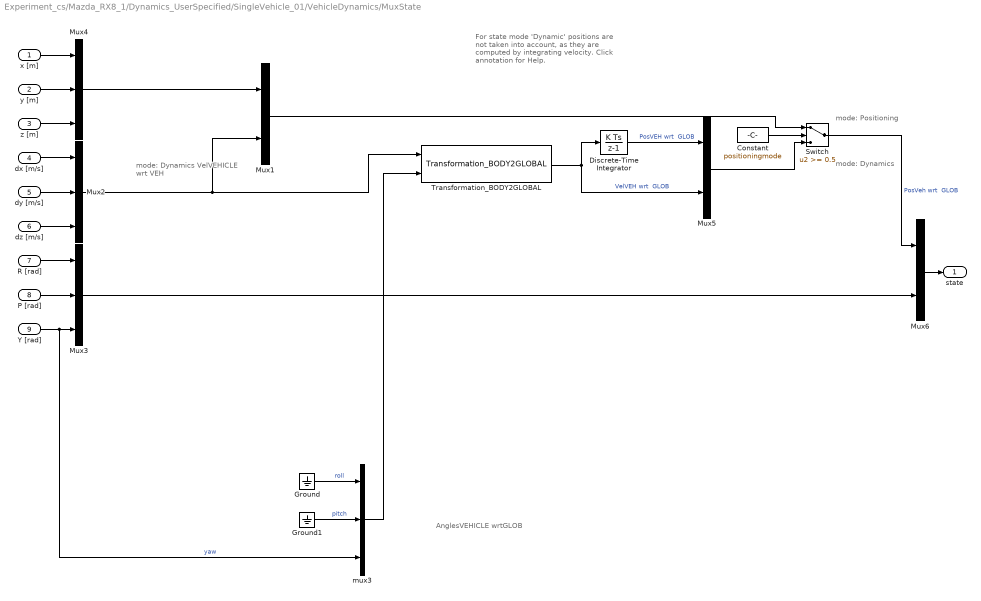
== system Experiment_cs/Mazda_RX8_1/Dynamics_UserSpecified/SingleVehicle_01/VehicleDynamics/MuxState ==
  note: For state mode 'Dynamic' positions
      | are not taken into account, as they
      | are computed by integrating velocity.
      | Click annotation for Help.
  note: AnglesVEHICLE
      | wrtGLOB
  note: mode: Dynamics
      | VelVEHICLE
      | wrt VEH
  note: mode: Positioning
  note: mode: Dynamics
  x [m] : Inport  SampleTime=TimeStep
  y [m] : Inport  Port=2  SampleTime=TimeStep
  z [m] : Inport  Port=3  SampleTime=TimeStep
  dx [m/s] : Inport  Port=4  SampleTime=TimeStep
  dy [m/s] : Inport  Port=5  SampleTime=TimeStep
  dz [m/s] : Inport  Port=6  SampleTime=TimeStep
  R [rad] : Inport  Port=7  SampleTime=TimeStep
  P [rad] : Inport  Port=8  SampleTime=TimeStep
  Y [rad] : Inport  Port=9  SampleTime=TimeStep
  Constant : Constant  DisableCoverage=on  Value=positioningmode
  Discrete-Time Integrator : DiscreteIntegrator  SampleTime=TimeStep  ICPrevOutput=DiscIntNeverNeededParam  ICPrevScaledInput=DiscIntNeverNeededParam
  Ground : Ground
  Ground1 : Ground
  Mux1 : Mux  Inputs=[3 3]
  Mux2 : Mux  Inputs=3
  Mux3 : Mux  Inputs=3
  Mux4 : Mux  Inputs=3
  Mux5 : Mux  Inputs=[3 3]
  Mux6 : Mux  Inputs=[6 3]
  Switch : Switch  Threshold=0.5
  Transformation_BODY2GLOBAL : PreScanSimulinkLibrary/Simple_Vehicle_Dynamics/Chassis/MuxDynState/Transformation_BODY2GLOBAL
  mux3 : Mux  Inputs=3
  state : Outport
  wires:
  Discrete-Time Integrator/1 -> Mux5/1  "PosVEH wrt  GLOB"
  Mux2/1 -> Transformation_BODY2GLOBAL/1, Mux1/2
  Ground/1 -> mux3/1  "roll"
  mux3/1 -> Transformation_BODY2GLOBAL/2
  Transformation_BODY2GLOBAL/1 -> Mux5/2, Discrete-Time Integrator/1  "VelVEH wrt  GLOB"
  Mux3/1 -> Mux6/2
  Y [rad]/1 -> Mux3/3, mux3/3  "yaw"
  Ground1/1 -> mux3/2  "pitch"
  x [m]/1 -> Mux4/1
  y [m]/1 -> Mux4/2
  z [m]/1 -> Mux4/3
  dx [m/s]/1 -> Mux2/1
  dy [m/s]/1 -> Mux2/2
  dz [m/s]/1 -> Mux2/3
  R [rad]/1 -> Mux3/1
  P [rad]/1 -> Mux3/2
  Switch/1 -> Mux6/1  "PosVeh wrt  GLOB"
  Mux1/1 -> Switch/1
  Mux5/1 -> Switch/3
  Mux4/1 -> Mux1/1
  Mux6/1 -> state/1
  Constant/1 -> Switch/2

== system Experiment_cs/Toyota_Yaris_1/Dynamics_UserSpecified/SingleVehicle_01/Controller/Actuation ==
  ArbitratedActuationReq : Inport
  ControllerMainBusIn : Inport  Port=2
  ActuatorDrivers : MATLAB Function  TreatAsAtomicUnit=on
  Bus Assignment : BusAssignment  AssignedSignals=ActuationCmdBus
  Bus Selector : BusSelector  OutputSignals=ActuationCmdBus
  DynamicControls : MATLAB Function  TreatAsAtomicUnit=on
  accelCmd : Outport
  brakeCmd : Outport  Port=2
  steerCmd : Outport  Port=3
  ControllerMainBusOut : Outport  Port=4
  wires:
  ActuatorDrivers/3(steering_cmd) -> steerCmd/1
  ActuatorDrivers/1(accel_cmd) -> accelCmd/1
  ActuatorDrivers/2(decel_cmd) -> brakeCmd/1
  Bus Assignment/1 -> ControllerMainBusOut/1
  DynamicControls/1(ActCmds) -> Bus Assignment/2, ActuatorDrivers/1(ActCmds)
  Bus Selector/1 -> DynamicControls/3(ActCmdsPrev)  "<ActuationCmdBus>"
  ArbitratedActuationReq/1 -> DynamicControls/1(ActReq)
  ControllerMainBusIn/1 -> Bus Selector/1, Bus Assignment/1, DynamicControls/2(Ctl)

== system Experiment_cs/Toyota_Yaris_1/Dynamics_UserSpecified/SingleVehicle_01/Controller/CollectSensorData ==
  PreScanSimData : Inport
  VehicleStateLast : Inport  Port=2
  ControllerMainBusIn : Inport  Port=3
  Bus Assignment : BusAssignment  AssignedSignals=FromPrescan,IdealSensors
  IdealSensorsProcess : Subsystem
  PrescanProcess : Subsystem
  PrescanSimDataBus : Outport
  IdealSensorBus : Outport  Port=2
  ControllerMainBusOut : Outport  Port=3
  wires:
  ControllerMainBusIn/1 -> Bus Assignment/1
  Bus Assignment/1 -> ControllerMainBusOut/1
  IdealSensorsProcess/1(IdealSensorsBus) -> Bus Assignment/3, IdealSensorBus/1
  VehicleStateLast/1 -> IdealSensorsProcess/1(VehicleState)
  PrescanProcess/1(PrescanSimDataBus) -> PrescanSimDataBus/1, Bus Assignment/2
  PreScanSimData/1 -> PrescanProcess/1(PrescanSimData)

== system Experiment_cs/Toyota_Yaris_1/Dynamics_UserSpecified/SingleVehicle_01/Controller/CtlMainBusUnitDelayAndInit ==
  CtlBus : Inport
  MATLAB Function : MATLAB Function  TreatAsAtomicUnit=on
  Memory : Memory  InheritSampleTime=on
  CtlBusDelayed : Outport
  wires:
  MATLAB Function/1(y) -> CtlBusDelayed/1
  CtlBus/1 -> Memory/1
  Memory/1 -> MATLAB Function/1(u)

== system Experiment_cs/Toyota_Yaris_1/Dynamics_UserSpecified/SingleVehicle_01/Controller/FeaturedFunctions ==
  SituationBus : Inport
  ControllerMainBusIn : Inport  Port=2
  Bus Assignment : BusAssignment  AssignedSignals=wpFollower
  Bus Assignment1 : BusAssignment  AssignedSignals=FunctionFeatures
  Bus Assignment2 : BusAssignment  AssignedSignals=situationBus
  Bus Selector : BusSelector  OutputSignals=FunctionFeatures
  Bus Selector2 : BusSelector  OutputSignals=FunctionFeatures.wpFollower
  wpFollower : MATLAB Function  TreatAsAtomicUnit=on
  FeatureReqBus : Outport
  ControllerMainBusOut : Outport  Port=2
  wires:
  Bus Selector2/1 -> wpFollower/1(prevWpAction)  "<wpFollower>"
  Bus Assignment2/1 -> ControllerMainBusOut/1
  wpFollower/2(newSituation) -> Bus Assignment2/2
  Bus Assignment1/1 -> Bus Assignment2/1
  Bus Assignment/1 -> FeatureReqBus/1, Bus Assignment1/2
  wpFollower/1(wpAction) -> Bus Assignment/2
  Bus Selector/1 -> Bus Assignment/1  "<FunctionFeatures>"
  SituationBus/1 -> wpFollower/2(prevSituation)
  ControllerMainBusIn/1 -> Bus Assignment1/1, Bus Selector2/1, Bus Selector/1

== system Experiment_cs/Toyota_Yaris_1/Dynamics_UserSpecified/SingleVehicle_01/Controller/SituationalAwareness ==
  PrescanSimDataBus : Inport
  IdealSensorBus : Inport  Port=2
  ControllerMainBusIn : Inport  Port=3
  Bus Assignment : BusAssignment  AssignedSignals=situationBus
  Bus Selector : BusSelector  OutputSignals=situationBus
  situationAwareness : MATLAB Function  TreatAsAtomicUnit=on
  SituationBus : Outport
  ControllerMainBusOut : Outport  Port=2
  wires:
  Bus Assignment/1 -> ControllerMainBusOut/1
  situationAwareness/1(newSituation) -> SituationBus/1, Bus Assignment/2
  IdealSensorBus/1 -> situationAwareness/3(idealSensors)
  PrescanSimDataBus/1 -> situationAwareness/2(prescanSimData)
  Bus Selector/1 -> situationAwareness/1(prevSituation)  "<situationBus>"
  ControllerMainBusIn/1 -> Bus Selector/1, Bus Assignment/1

== system Experiment_cs/Toyota_Yaris_1/Dynamics_UserSpecified/SingleVehicle_01/Controller/StrategicArbitration ==
  FeatureReqBus : Inport
  ControllerMainBusIn : Inport  Port=2
  Arbitration : MATLAB Function  TreatAsAtomicUnit=on
  Bus Assignment : BusAssignment  AssignedSignals=ArbitratedActuationReq
  ArbitratedActuationReq : Outport
  ControllerMainBusOut : Outport  Port=2
  wires:
  Bus Assignment/1 -> ControllerMainBusOut/1
  Arbitration/1(ArbitratedReq) -> ArbitratedActuationReq/1, Bus Assignment/2
  FeatureReqBus/1 -> Arbitration/1(FunctionFeatures)
  ControllerMainBusIn/1 -> Bus Assignment/1

== system Experiment_cs/Toyota_Yaris_1/Dynamics_UserSpecified/SingleVehicle_01/Monitor/ControllerMainBusStorage ==
  ControllerMainBus : Inport
  ArbitratedActuationReqStorage : ToWorkspace  VariableName=vd02_DataControllerMain_ArbitrationActuationReq  SaveFormat=Timeseries  SampleTime=-1
  Bus Selector : BusSelector  OutputSignals=ArbitratedActuationReq,FunctionFeatures.wpFollower,situationBus.wP.finalWayPoint,situationBus.wP.currentWayPoint,situationBus.wP.wayPointArray,situationBus.selfAwarenessBus,IdealSensors,FromPrescan
  FromPrescanStorage : ToWorkspace  VariableName=vd02_DataControllerMain_FromPrescan  SaveFormat=Timeseries  SampleTime=-1
  Ground_1 : Ground
  IdealSensorsStorage : ToWorkspace  VariableName=vd02_DataControllerMain_IdealSensors  SaveFormat=Timeseries  SampleTime=-1
  Terminator_1 : Terminator
  currentWayPointStorage : ToWorkspace  VariableName=vd02_DataControllerMain_currentWayPoint  SaveFormat=Timeseries  SampleTime=-1
  finalWayPointStorarge : ToWorkspace  VariableName=vd02_DataControllerMain_finalWayPoint  SaveFormat=Timeseries  SampleTime=-1
  selfAwareessBusStorage : ToWorkspace  VariableName=vd02_DataControllerMain_selfAwareessBus  SaveFormat=Timeseries  SampleTime=-1
  wayPointArrayStorage : ToWorkspace  VariableName=vd02_DataControllerMain_wayPointArray  SampleTime=-1
  wpFollowerStorage : ToWorkspace  VariableName=vd02_DataControllerMain_wpFollower  SaveFormat=Timeseries  SampleTime=-1
  wires:
  Bus Selector/7 -> IdealSensorsStorage/1  "<IdealSensors>"
  Bus Selector/4 -> currentWayPointStorage/1  "<currentWayPoint>"
  Bus Selector/6 -> selfAwareessBusStorage/1  "<selfAwarenessBus>"
  Bus Selector/8 -> FromPrescanStorage/1  "<FromPrescan>"
  Bus Selector/3 -> finalWayPointStorarge/1  "<finalWayPoint>"
  Bus Selector/2 -> wpFollowerStorage/1  "<wpFollower>"
  Bus Selector/1 -> ArbitratedActuationReqStorage/1  "<ArbitratedActuationReq>"
  ControllerMainBus/1 -> Bus Selector/1
  Bus Selector/5 -> Terminator_1/1  "<wayPointArray>"
  Ground_1/1 -> wayPointArrayStorage/1

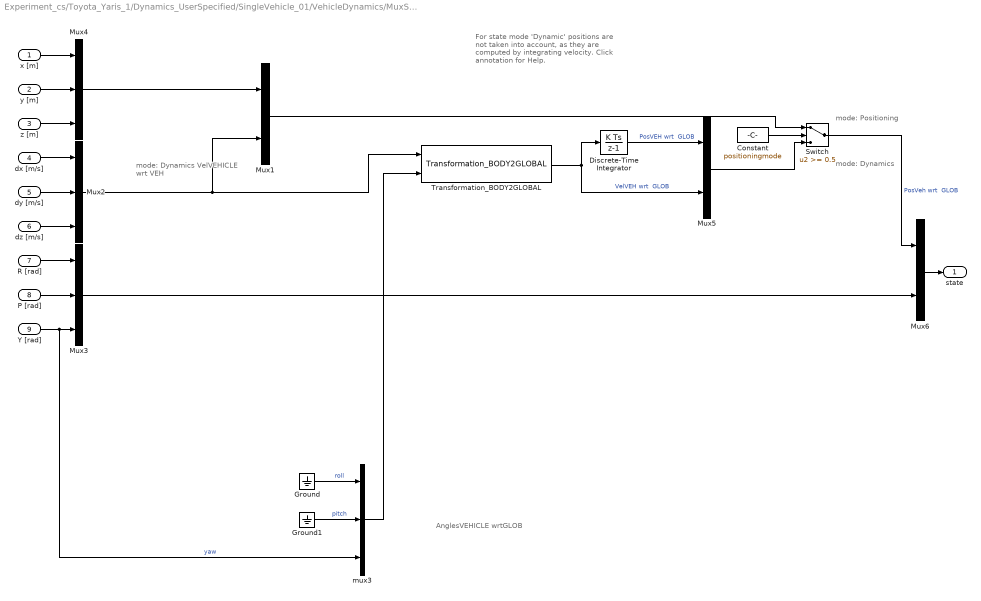
== system Experiment_cs/Toyota_Yaris_1/Dynamics_UserSpecified/SingleVehicle_01/VehicleDynamics/MuxState ==
  note: For state mode 'Dynamic' positions
      | are not taken into account, as they
      | are computed by integrating velocity.
      | Click annotation for Help.
  note: AnglesVEHICLE
      | wrtGLOB
  note: mode: Dynamics
      | VelVEHICLE
      | wrt VEH
  note: mode: Positioning
  note: mode: Dynamics
  x [m] : Inport  SampleTime=TimeStep
  y [m] : Inport  Port=2  SampleTime=TimeStep
  z [m] : Inport  Port=3  SampleTime=TimeStep
  dx [m/s] : Inport  Port=4  SampleTime=TimeStep
  dy [m/s] : Inport  Port=5  SampleTime=TimeStep
  dz [m/s] : Inport  Port=6  SampleTime=TimeStep
  R [rad] : Inport  Port=7  SampleTime=TimeStep
  P [rad] : Inport  Port=8  SampleTime=TimeStep
  Y [rad] : Inport  Port=9  SampleTime=TimeStep
  Constant : Constant  DisableCoverage=on  Value=positioningmode
  Discrete-Time Integrator : DiscreteIntegrator  SampleTime=TimeStep  ICPrevOutput=DiscIntNeverNeededParam  ICPrevScaledInput=DiscIntNeverNeededParam
  Ground : Ground
  Ground1 : Ground
  Mux1 : Mux  Inputs=[3 3]
  Mux2 : Mux  Inputs=3
  Mux3 : Mux  Inputs=3
  Mux4 : Mux  Inputs=3
  Mux5 : Mux  Inputs=[3 3]
  Mux6 : Mux  Inputs=[6 3]
  Switch : Switch  Threshold=0.5
  Transformation_BODY2GLOBAL : PreScanSimulinkLibrary/Simple_Vehicle_Dynamics/Chassis/MuxDynState/Transformation_BODY2GLOBAL
  mux3 : Mux  Inputs=3
  state : Outport
  wires:
  Discrete-Time Integrator/1 -> Mux5/1  "PosVEH wrt  GLOB"
  Mux2/1 -> Transformation_BODY2GLOBAL/1, Mux1/2
  Ground/1 -> mux3/1  "roll"
  mux3/1 -> Transformation_BODY2GLOBAL/2
  Transformation_BODY2GLOBAL/1 -> Mux5/2, Discrete-Time Integrator/1  "VelVEH wrt  GLOB"
  Mux3/1 -> Mux6/2
  Y [rad]/1 -> Mux3/3, mux3/3  "yaw"
  Ground1/1 -> mux3/2  "pitch"
  x [m]/1 -> Mux4/1
  y [m]/1 -> Mux4/2
  z [m]/1 -> Mux4/3
  dx [m/s]/1 -> Mux2/1
  dy [m/s]/1 -> Mux2/2
  dz [m/s]/1 -> Mux2/3
  R [rad]/1 -> Mux3/1
  P [rad]/1 -> Mux3/2
  Switch/1 -> Mux6/1  "PosVeh wrt  GLOB"
  Mux1/1 -> Switch/1
  Mux5/1 -> Switch/3
  Mux4/1 -> Mux1/1
  Mux6/1 -> state/1
  Constant/1 -> Switch/2

== system Experiment_cs/Actros_2541_1/Dynamics_UserSpecified/SingleVehicle_01/Controller/CollectSensorData/IdealSensorsProcess ==
  VehicleState : Inport
  Bus Creator : BusCreator  Inputs=12  OutDataTypeStr=Bus: VehState
  Bus Selector : BusSelector  OutputSignals=x,y,z,theta,phi,psi,u,v,w,dtheta,dphi,dpsi
  IdealSensorsBus : Outport
  wires:
  Bus Creator/1 -> IdealSensorsBus/1
  Bus Selector/3 -> Bus Creator/3  "<z>"
  Bus Selector/12 -> Bus Creator/12  "<dpsi>"
  Bus Selector/5 -> Bus Creator/5  "<phi>"
  Bus Selector/2 -> Bus Creator/2  "<y>"
  Bus Selector/9 -> Bus Creator/9  "<w>"
  Bus Selector/4 -> Bus Creator/4  "<theta>"
  Bus Selector/6 -> Bus Creator/6  "<psi>"
  Bus Selector/11 -> Bus Creator/11  "<dphi>"
  Bus Selector/10 -> Bus Creator/10  "<dtheta>"
  Bus Selector/7 -> Bus Creator/7  "<u>"
  Bus Selector/8 -> Bus Creator/8  "<v>"
  Bus Selector/1 -> Bus Creator/1  "<x>"
  VehicleState/1 -> Bus Selector/1

== system Experiment_cs/Actros_2541_1/Dynamics_UserSpecified/SingleVehicle_01/Controller/CollectSensorData/PrescanProcess ==
  PrescanSimData : Inport
  Bus Creator : BusCreator  Inputs=12  OutDataTypeStr=Bus: PrescanSimData
      settings: InheritFromInputs=off
  SELF_Demux : Subsystem  Tag=DemuxSELF  mask(PreScan Demux Block:){}
      settings: DeleteFcn=PreScanBlockDeleteFcn;
      mask Display:
      | port_label('output',1,'x [m]')
      | port_label('output',2,'y [m]')
      | port_label('output',3,'z [m]','texmode','on')
      | port_label('output',4,'Rotx [deg]','texmode','on')
      | port_label('output',5,'Roty [deg]','texmode','on')
      | port_label('output',6,'Rotz [deg]','texmode','on')
      | port_label('output',7,'GPS lat [deg]','texmode','on')
      | port_label('output',8,'GPS long [deg]','texmode','on')
      | port_label('output',9,'GPS alt [m]','texmode','on')
      | port_label('output',10,'Velocity [m/s]')
      | port_label('output',11,'Heading [deg]')
      | port_label('output',12,'Yaw rate [deg/s]')
  PrescanSimDataBus : Outport
  wires:
  SELF_Demux/12(yaw rate [deg/s]) -> Bus Creator/12  "Yaw_rate"
  SELF_Demux/11(heading [deg]) -> Bus Creator/11  "heading"
  SELF_Demux/7(GPS lat [deg]) -> Bus Creator/7  "GPS_lat"
  SELF_Demux/6(rotz [deg]) -> Bus Creator/6  "Rotz"
  SELF_Demux/10(velocity [m/s]) -> Bus Creator/10  "u"
  SELF_Demux/8(GPS long [deg]) -> Bus Creator/8  "GPS_long"
  SELF_Demux/9(GPS alt [m]) -> Bus Creator/9  "GPS_alt"
  SELF_Demux/5(roty [deg]) -> Bus Creator/5  "Roty"
  SELF_Demux/4(rotx [deg]) -> Bus Creator/4  "Rotx"
  SELF_Demux/3(z [m]) -> Bus Creator/3  "z"
  SELF_Demux/2(y [m]) -> Bus Creator/2  "y"
  Bus Creator/1 -> PrescanSimDataBus/1
  PrescanSimData/1 -> SELF_Demux/1(SELF)
  SELF_Demux/1(x [m]) -> Bus Creator/1  "x"

== system Experiment_cs/Audi_A8_1/Dynamics_UserSpecified/SingleVehicle_01/Controller/CollectSensorData/IdealSensorsProcess ==
  VehicleState : Inport
  Bus Creator : BusCreator  Inputs=12  OutDataTypeStr=Bus: VehState
  Bus Selector : BusSelector  OutputSignals=x,y,z,theta,phi,psi,u,v,w,dtheta,dphi,dpsi
  IdealSensorsBus : Outport
  wires:
  Bus Creator/1 -> IdealSensorsBus/1
  Bus Selector/3 -> Bus Creator/3  "<z>"
  Bus Selector/12 -> Bus Creator/12  "<dpsi>"
  Bus Selector/5 -> Bus Creator/5  "<phi>"
  Bus Selector/2 -> Bus Creator/2  "<y>"
  Bus Selector/9 -> Bus Creator/9  "<w>"
  Bus Selector/4 -> Bus Creator/4  "<theta>"
  Bus Selector/6 -> Bus Creator/6  "<psi>"
  Bus Selector/11 -> Bus Creator/11  "<dphi>"
  Bus Selector/10 -> Bus Creator/10  "<dtheta>"
  Bus Selector/7 -> Bus Creator/7  "<u>"
  Bus Selector/8 -> Bus Creator/8  "<v>"
  Bus Selector/1 -> Bus Creator/1  "<x>"
  VehicleState/1 -> Bus Selector/1
